simulink model "rtwdemo_slbus"  (Simulink 6.0)
settings: Solver=FixedStepDiscrete  StartTime=0.0  StopTime=10.0  FixedStep=1  RelTol=1e-3
PostLoadFcn:
  | rtwdemo_slbus_data
libraries: rtwdemowidgets x3
settings Model: Creator=The MathWorks Inc.  LastModifiedBy=batserve  ExtModeAutoUpdateStatusClock=off
settings DataIOCC: SaveOutput=off  SaveTime=off
settings OptimizationCC: InlineParams=on  EnforceIntegerDowncast=off  ExpressionFolding=off  StateBitsets=on  DataBitsets=on  UseTempVars=on
settings DebuggingCC: CheckExecutionContextPreStartOutputMsg=on  CheckExecutionContextRuntimeOutputMsg=on
settings RTWCC: Description=RTW Embedded Coder (no auto configuration)  GenerateReport=on  RTWVerbose=off  ProcessScript=grt_make_rtw_hook  LaunchReport=on
settings CodeAppCC: ForceParamTrailComments=on
settings GRTTargetCC: MatFileLogging=off

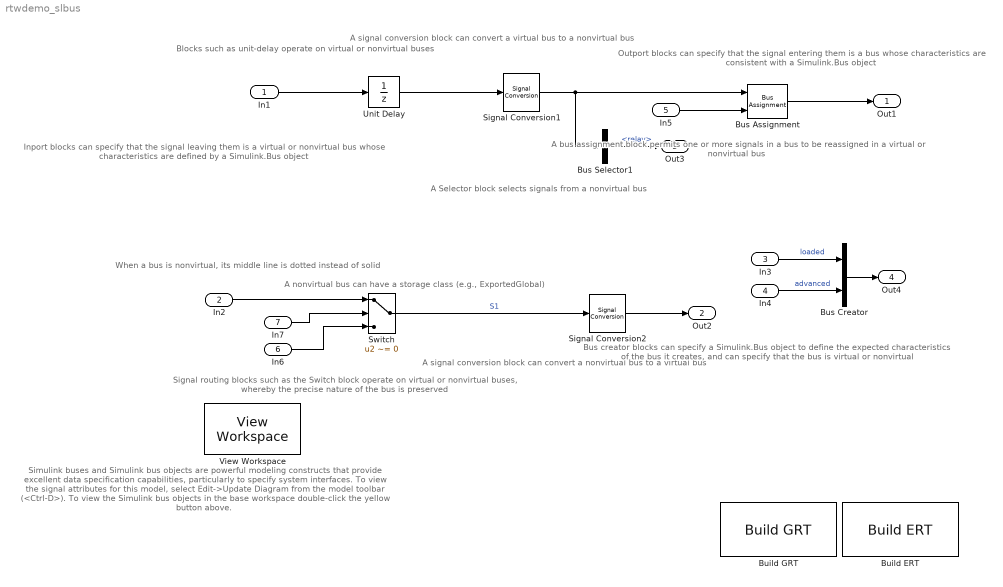
== system rtwdemo_slbus ==
  note: Blocks such as unit-delay operate
      | on virtual or nonvirtual buses
  note: A signal conversion block  can convert
      | a virtual bus to a nonvirtual bus
  note: A bus assignment block permits one or
      | more signals in a bus to be reassigned
      | in a virtual or nonvirtual bus
  note: Outport blocks can specify that
      | the signal entering them is a bus
      | whose characteristics are consistent
      | with a Simulink.Bus object
  note: Inport blocks can specify that
      | the signal leaving them is a
      | virtual or nonvirtual bus whose
      | characteristics are defined by a
      | Simulink.Bus object
  note: Signal routing blocks such
      | as the Switch block operate
      | on virtual or nonvirtual buses,
      | whereby the precise nature
      | of the bus is preserved
  note: A signal conversion block
      | can convert a nonvirtual
      | bus to a virtual bus
  note: A Selector block selects signals
      | from a nonvirtual bus
  note: When a bus is
      | nonvirtual, its middle line
      | is dotted instead of solid
  note: A nonvirtual bus can have a storage
      | class (e.g., ExportedGlobal)
  note: Simulink buses and Simulink bus objects are powerful modeling constructs that provide
      | excellent data specification capabilities, particularly to specify system interfaces.
      |
      | To view the signal attributes for this model, select Edit->Update Diagram from the
      | model toolbar (<Ctrl-D>).  To view the Simulink bus objects in the base workspace
      | double-click the yellow button above.
  note: Bus creator blocks can specify
      | a Simulink.Bus object to define the
      | expected characteristics of the bus it
      | creates, and can specify that the
      | bus is virtual or nonvirtual
  In1 : Inport  Port=1  UseBusObject=on  LatchInput=off
      settings: BusObject=BusObject1
  In2 : Inport  Port=2  UseBusObject=on  LatchInput=off  BusOutputAsStruct=on
  In3 : Inport  Port=3  DataType=boolean  LatchInput=off
  In4 : Inport  Port=4  DataType=boolean  LatchInput=off
  In5 : Inport  Port=5  DataType=boolean  LatchInput=off
  In6 : Inport  Port=6  UseBusObject=on  LatchInput=off  BusOutputAsStruct=on
  In7 : Inport  Port=7  DataType=boolean  LatchInput=off
  Build ERT : rtwdemowidgets/Build ERT  attrib_overrides={}
  Build GRT : rtwdemowidgets/Build GRT  attrib_overrides={}
  Bus Creator : BusCreator  DialogController=Simulink.DDGSource_Bus  Inputs=2  UseBusObject=on  NonVirtualBus=on
      settings: BusObject=BusObject2
  Bus Selector1 : BusSelector  DialogController=Simulink.DDGSource_Bus  OutputSignals=relay
  Bus Assignment : BusAssignment  DialogController=Simulink.DDGSource_Bus  AssignedSignals=relay
  Signal Conversion1 : SignalConversion  ConversionOutput=Nonvirtual bus
  Signal Conversion2 : SignalConversion  ConversionOutput=Virtual bus
  Switch : Switch  Criteria=u2 ~= 0  ZeroCross=off
  Unit Delay : UnitDelay
  View Workspace : rtwdemowidgets/View Workspace
  Out1 : Outport  UseBusObject=on
      settings: BusObject=BusObject1
  Out2 : Outport  Port=2  UseBusObject=on
  Out3 : Outport  Port=3
  Out4 : Outport  Port=4  UseBusObject=on
      settings: BusObject=BusObject2
  wires:
  In1/1 -> Unit Delay/1
  Unit Delay/1 -> Signal Conversion1/1
  In2/1 -> Switch/1
  Switch/1 -> Signal Conversion2/1  "S1"
  Signal Conversion2/1 -> Out2/1
  Bus Selector1/1 -> Out3/1  "<relay>"
  Signal Conversion1/1 -> Bus Assignment/1, Bus Selector1/1
  Bus Assignment/1 -> Out1/1
  In5/1 -> Bus Assignment/2
  In6/1 -> Switch/3
  In7/1 -> Switch/2
  In3/1 -> Bus Creator/1  "loaded"
  In4/1 -> Bus Creator/2  "advanced"
  Bus Creator/1 -> Out4/1
